simulink library "Lib_HeatXfer_0DtransconductionLS_TMATS"  (R2019b)
settings: Solver=ode45  StartTime=0.0  StopTime=10.0  RelTol=1e-3  EnableMultiTasking=on
Description:
  | Thomas Modules
settings Model: Creator=jwchapm2  LastModifiedBy=bhisma
settings DataIOCC: LimitDataPoints=on  SaveFormat=Array  ReturnWorkspaceOutputs=off
settings OptimizationCC: ExpressionDepthLimit=2147483647  LifeSpan=inf
settings DebuggingCC: UnderspecifiedInitializationDetection=Classic  MergeDetectMultiDrivingBlocksExec=none  SolverPrmCheckMsg=warning  StateNameClashWarn=warning  SFUnexpectedBacktrackingDiag=warning  SFNoUnconditionalDefaultTransitionDiag=warning  SFExecutionAtInitializationDiag=none  ArithmeticOperatorsInVariantConditions=warning
settings HardwareCC: ProdBitPerPointer=32  ProdBitPerSizeT=32  ProdBitPerPtrDiffT=32  ProdLargestAtomicFloat=None  ProdIntDivRoundTo=Undefined  ProdEndianess=Unspecified  ProdWordSize=32  ProdHWDeviceType=32-bit Generic
settings ModelReferenceCC: PropagateSignalLabelsOutOfModel=off
settings SFSimCC: SimUseLocalCustomCode=off  CustomCodeUndefinedFunction=UseInterfaceOnly
settings RTWCC: RTWUseLocalCustomCode=off
settings CodeAppCC: StateflowObjectComments=on
settings GRTTargetCC: TargetLangStandard=C89/C90 (ANSI)  GeneratePreprocessorConditionals=Disable all
settings ConfigComp: CovMetricSettings=dw  CovHtmlReporting=on  CovSaveCumulativeToWorkspaceVar=on  CovSaveSingleToWorkspaceVar=on  CovExternalEMLEnable=off

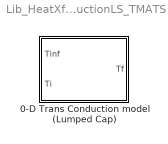
== system Lib_HeatXfer_0DtransconductionLS_TMATS ==
  0-D Trans Conduction model (Lumped Cap) : Subsystem  mask(T-MATS: 0-D Trans Conduction model (Lumped Cap) Block){dt_M=1, h_M=1, k_M=1, rho_M=2, c_M=3, L_M=4, BlkNm_M=double(gcb)}
      mask prompts: dt_M "Time Step (dt)"; h_M "convection heat transfer coefficient (h)"; k_M "thermal conductivity (k)"; rho_M "mass density (rho)"; c_M "specific heat (c)"; L_M "characteristic length (L = V/A)"; BlkNm_M "block name"
      mask help:
      | This function models the transient conduction of a lumped system via the lumped capacitance method.
      |
      | Export values are calculated based on a single time step. If additional dynamic behavior is required a simulink memory block may be used to update the temperature initial conditions.
      mask Help: web(which('HeatXfer_TMATS_0DTCondLS.html'),'-helpbrowser')

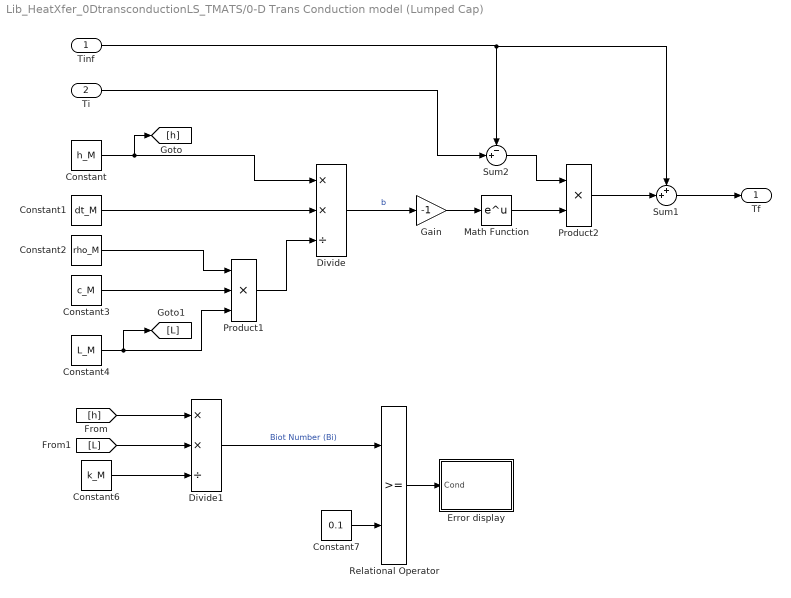
== system Lib_HeatXfer_0DtransconductionLS_TMATS/0-D Trans Conduction model (Lumped Cap) ==
  Tinf : Inport
  Ti : Inport  Port=2
  Constant : Constant  Value=h_M
  Constant1 : Constant  Value=dt_M
  Constant2 : Constant  Value=rho_M
  Constant3 : Constant  Value=c_M
  Constant4 : Constant  Value=L_M
  Constant6 : Constant  Value=k_M
  Constant7 : Constant  Value=0.1
  Divide : Product  Inputs=**/
  Divide1 : Product  Inputs=**/
  Error display : MATLAB Function  TreatAsAtomicUnit=on
  Gain : Gain  Gain=-1
  Math Function : Math  SaturateOnIntegerOverflow=on
  Product1 : Product  Inputs=3
  Product2 : Product
  Relational Operator : RelationalOperator  OutDataTypeStr=boolean  RndMeth=Nearest
  Sum1 : Sum  Inputs=++|
  Sum2 : Sum  Inputs=-+|
  Tf : Outport
  wires:
  Constant1/1 -> Divide/2
  Relational Operator/1 -> Error display/1(Cond)
  Ti/1 -> Sum2/2
  Sum2/1 -> Product2/1
  Gain/1 -> Math Function/1
  Sum1/1 -> Tf/1
  Product2/1 -> Sum1/2
  Tinf/1 -> Sum2/1, Sum1/1
  Math Function/1 -> Product2/2
  Constant/1 -> [h], Divide/1
  Product1/1 -> Divide/3
  Constant4/1 -> [L], Product1/3
  Constant2/1 -> Product1/1
  Divide/1 -> Gain/1  "b"
  Constant3/1 -> Product1/2
  Constant6/1 -> Divide1/3
  [L] -> Divide1/2
  [h] -> Divide1/1
  Divide1/1 -> Relational Operator/1  "Biot Number (Bi)"
  Constant7/1 -> Relational Operator/2

== matlab function Lib_HeatXfer_0DtransconductionLS_TMATS/0-D Trans Conduction model (Lumped Cap)/Error display ==
  data: Cond input; BlkNm_M parameter
function fcn(Cond,BlkNm_M)
%Error message
% check to determine if lumped capacitance method is appropriate
if Cond == 1
    disp(['Error in block ', BlkNm_M,', Bi <= 0.1 , input properties not appropriate for modeling method']); 
end
